simulink model "pratica13S"  (R2021b)
settings: Solver=VariableStepAuto  StartTime=0.0  StopTime=10.0  RelTol=1e-3
values from neighbouring files (symbols this model uses):
  Fl = [0.5357 -0.2329 0 ; 0.1950 0.9666 0 ; 0 -1.1946 1]    [pratica13.m]
  Hl = [0.1950 ; 0.0279 ; 0]    [pratica13.m]
  K = place(Fl, Hl, Pd)    [pratica13.m]
  R = 1.15    [pratica13.m]
  T0 = (2*pi)/ws    [pratica13.m]
undefined symbols (not defined in the file or in its folder): Dc
settings Model: Creator=carlo  LastModifiedBy=carlo

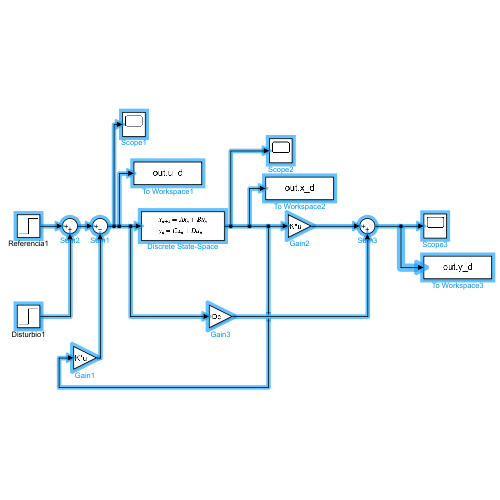
[thumbnail: Simulink's stored preview of the top-level diagram]
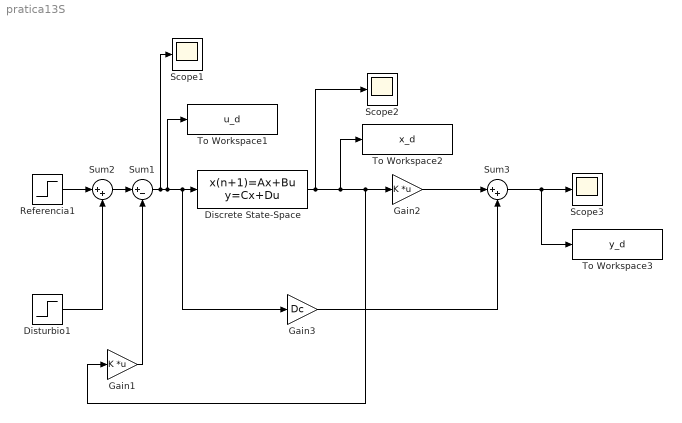
== system pratica13S ==
  Discrete State-Space : DiscreteStateSpace  A=Fl  B=Hl  C=[1 0 0 ; 0 1 0 ; 0 0 1]  D=[0 ; 0 ; 0]  SampleTime=T0
  Disturbio1 : Step  Time=12  After=R  SampleTime=0
  Gain1 : Gain  Gain=K  Multiplication=Matrix(K*u)
  Gain2 : Gain  Gain=K  Multiplication=Matrix(K*u)
  Gain3 : Gain  Gain=Dc
  Referencia1 : Step  Time=0  After=R  SampleTime=0
  Scope1 : Scope
  Scope2 : Scope
  Scope3 : Scope
  Sum1 : Sum  Inputs=|+-
  Sum2 : Sum  Inputs=|++
  Sum3 : Sum  Inputs=|++
  To Workspace1 : ToWorkspace  VariableName=u_d  SaveFormat=Timeseries  SampleTime=-1
  To Workspace2 : ToWorkspace  VariableName=x_d  SaveFormat=Timeseries  SampleTime=-1
  To Workspace3 : ToWorkspace  VariableName=y_d  SaveFormat=Timeseries  SampleTime=-1
  wires:
  Sum1/1 -> Scope1/1, To Workspace1/1, Gain3/1, Discrete State-Space/1
  Gain1/1 -> Sum1/2
  Gain2/1 -> Sum3/1
  Discrete State-Space/1 -> Scope2/1, To Workspace2/1, Gain1/1, Gain2/1
  Referencia1/1 -> Sum2/1
  Sum2/1 -> Sum1/1
  Gain3/1 -> Sum3/2
  Disturbio1/1 -> Sum2/2
  Sum3/1 -> To Workspace3/1, Scope3/1
